simulink model "Consensus_Animation"  (R2020a)
settings: Solver=VariableStepAuto  StartTime=0.0  StopTime=t_simulation  RelTol=1e-3
libraries: vrlib x5
settings Model: Creator=andre  LastModifiedBy=andre

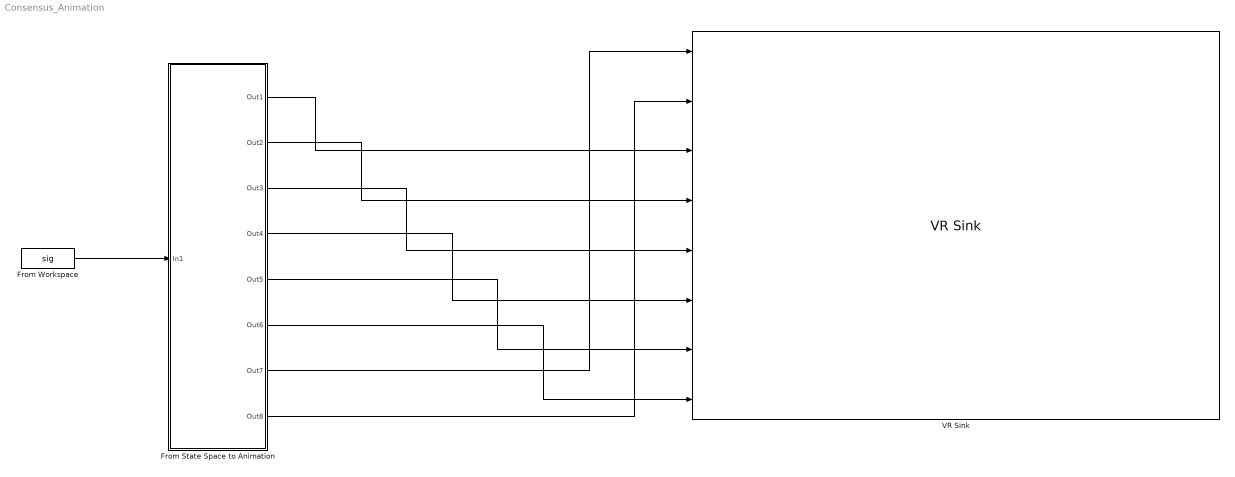
== system Consensus_Animation ==
  From Workspace : FromWorkspace  VariableName=sig
  From State Space to Animation : Subsystem
  VR Sink : vrlib/VR Sink  InstantiateOnLoad=on  SampleTime=0.01  ViewEnable=on  RemoteChange=off  RemoteView=off  FieldsWritten=Unicycle_4.rotation.4.1.1.double#Unicycle_4.translation.3.1.1.double#Unicycle_1.rotation.4.1.1.double#Unicycle_1.translation.3.1.1.double#Unicycle_2.rotation.4.1.1.double#Unicycle_2.translation.3.1.1.double#Unicycle_3.rotation.4.1.1.double#Unicycle_3.translation.3.1.1.double  WorldFileName=Consensus Animation.WRL  AutoView=off  VideoDimensions=[]  AllowVariableSize=off
  wires:
  From Workspace/1 -> From State Space to Animation/1(In1)
  From State Space to Animation/1(Out1) -> VR Sink/3
  From State Space to Animation/2(Out2) -> VR Sink/4
  From State Space to Animation/3(Out3) -> VR Sink/5
  From State Space to Animation/4(Out4) -> VR Sink/6
  From State Space to Animation/5(Out5) -> VR Sink/7
  From State Space to Animation/6(Out6) -> VR Sink/8
  From State Space to Animation/7(Out7) -> VR Sink/1
  From State Space to Animation/8(Out8) -> VR Sink/2

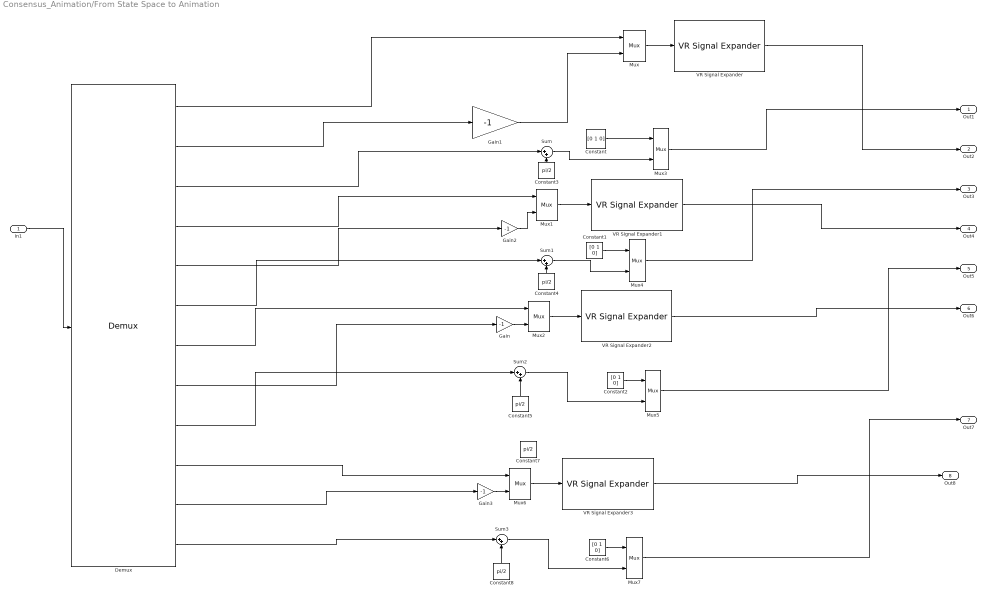
== system Consensus_Animation/From State Space to Animation ==
  In1 : Inport
  Constant{,1..2,6} (4 alike) : Constant  Value=[0 1 0]
  Constant{3..5,7..8} (5 alike) : Constant  Value=pi/2
  Demux : Demux  Outputs=12
  Gain{,1..3} (4 alike) : Gain  Gain=-1
  Mux{,1..7} (8 alike) : Mux  Inputs=2
  Sum{,1..3} (4 alike) : Sum  Inputs=|++
  VR Signal Expander{,1..3} (4 alike) : vrlib/VR Signal Expander  outwidth=3  outidx=[1 3]
  Out1 : Outport
  Out2 : Outport  Port=2
  Out3 : Outport  Port=3
  Out4 : Outport  Port=4
  Out5 : Outport  Port=5
  Out6 : Outport  Port=6
  Out7 : Outport  Port=7
  Out8 : Outport  Port=8
  wires:
  Constant1/1 -> Mux4/1
  Mux/1 -> VR Signal Expander/1
  Gain1/1 -> Mux/2
  Mux5/1 -> Out5/1
  Constant/1 -> Mux3/1
  Demux/2 -> Gain1/1
  Gain/1 -> Mux2/2
  Constant2/1 -> Mux5/1
  Mux1/1 -> VR Signal Expander1/1
  Mux2/1 -> VR Signal Expander2/1
  Demux/7 -> Mux2/1
  Demux/4 -> Mux1/1
  Demux/8 -> Gain/1
  Gain2/1 -> Mux1/2
  Demux/1 -> Mux/1
  Demux/5 -> Gain2/1
  In1/1 -> Demux/1
  Mux4/1 -> Out3/1
  VR Signal Expander/1 -> Out2/1
  Mux3/1 -> Out1/1
  VR Signal Expander1/1 -> Out4/1
  VR Signal Expander2/1 -> Out6/1
  Constant3/1 -> Sum/2
  Sum/1 -> Mux3/2
  Constant4/1 -> Sum1/2
  Sum1/1 -> Mux4/2
  Constant5/1 -> Sum2/2
  Sum2/1 -> Mux5/2
  Demux/3 -> Sum/1
  Demux/6 -> Sum1/1
  Demux/9 -> Sum2/1
  VR Signal Expander3/1 -> Out8/1
  Gain3/1 -> Mux6/2
  Mux6/1 -> VR Signal Expander3/1
  Constant6/1 -> Mux7/1
  Sum3/1 -> Mux7/2
  Mux7/1 -> Out7/1
  Constant8/1 -> Sum3/2
  Demux/10 -> Mux6/1
  Demux/11 -> Gain3/1
  Demux/12 -> Sum3/1
